simulink library "Controller_Bang_Bang"  (Simulink 8.2)
settings: Solver=ode45  StartTime=0.0  StopTime=10.0  RelTol=1e-3
settings Model: Creator=lena.frank  LastModifiedBy=drhf

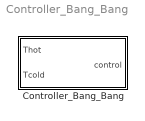
== system Controller_Bang_Bang ==
  Controller_Bang_Bang : Subsystem  mask(bang bang controler){deltaTon=5, deltaToff=1, Tmax=95}
      mask prompts: deltaTon "deltaT-on [K]"; deltaToff "deltaT-off [K]"; Tmax "maximum temperature [degree centigrade]"
      mask help:
      | Hysteresis controller for thermal systems. Output is set to zero if Thot or Tcold is bigger than Tmax.
      | deltaT = Thot - Tcold
      mask Help: web(fullfile(path_carnot('help'),'Controller_Bang_Bang.html'),'-helpbrowser')
      mask Display: plot(-30,0,150,100,[70,100,40,10,70,70,10,10],[50,80,80,50,50,20,20,50],[100,70],[50,20],[20,50,50,20,20],[40,40,30,30,40],[62,62,62,61,59,58,58,60],[42,41,39,38,38,40,42,43],[61,62,62,61,60,59,58,58,58,59],[32,31,30,28,27,28,28,30,31,32])

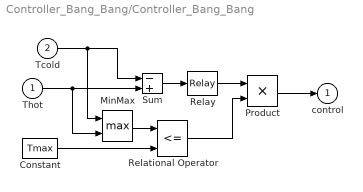
== system Controller_Bang_Bang/Controller_Bang_Bang ==
  Thot : Inport
  Tcold : Inport  Port=2
  Constant : Constant  Value=Tmax
  MinMax : MinMax  Function=max  Inputs=2  SaturateOnIntegerOverflow=on  InputSameDT=on
  Product : Product  OutDataTypeStr=double  SaturateOnIntegerOverflow=on
  Relational Operator : RelationalOperator  Operator=<=  InputSameDT=on
  Relay : Relay  OnSwitchValue=deltaTon  OffSwitchValue=deltaToff
  Sum : Sum  Inputs=-+  SaturateOnIntegerOverflow=on  InputSameDT=on  OutDataTypeStr=Inherit: Same as first input
  control : Outport
  wires:
  Relational Operator/1 -> Product/2
  Product/1 -> control/1
  Relay/1 -> Product/1
  MinMax/1 -> Relational Operator/1
  Tcold/1 -> MinMax/1, Sum/1
  Thot/1 -> MinMax/2, Sum/2
  Constant/1 -> Relational Operator/2
  Sum/1 -> Relay/1
